simulink model "mcbdemo_28035_TARGET"  (R2021a)
settings: Solver=FixedStepDiscrete  StartTime=0.0  StopTime=4  RelTol=1e-3  EnableMultiTasking=on
InitFcn:
  | mcb_28035_parameters;
values from neighbouring files (symbols this model uses):
  Gain = 10    [mcb_28035_parameters.m]
  T_pwm = 1/PWM_frequency    (= 0.0001)    [mcb_28035_parameters.m]
  Ts = T_pwm    (= 0.0001)    [mcb_28035_parameters.m]
  Ts_inverter = T_pwm/2    (= 5e-05)    [mcb_28035_parameters.m]
  Ts_motor = T_pwm/2    (= 5e-05)    [mcb_28035_parameters.m]
  Ts_simulink = T_pwm/2    (= 5e-05)    [mcb_28035_parameters.m]
undefined symbols (not defined in the file or in its folder): DiscIntNeverNeededParam, Down, GPTRIP1SEL, GPTRIP2SEL, inverter, PI_params, pmsm, target, TZ1, TZ2, Up
libraries: mcbcontrolslib x20, simulink x11, c2802xlib x9, tiiqmathlib x5, c2803xlib x5, mcbpositiondecoderlib x3, c280xlib x2, dspsigops x1, c2000lib x1, autolibpmsmexterior x1
(part 2 of 2)

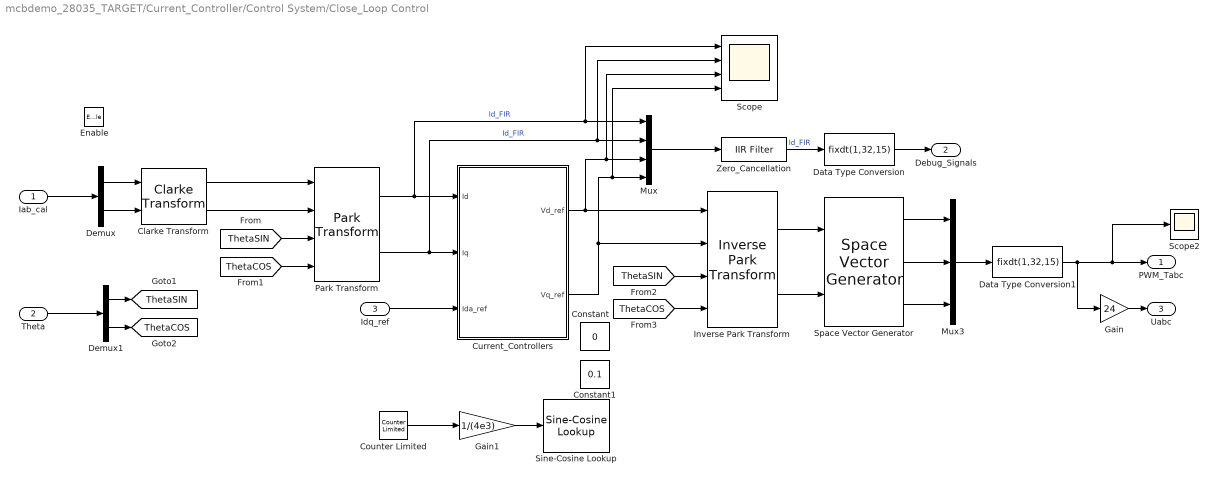
== system mcbdemo_28035_TARGET/Current_Controller/Control System/Close_Loop Control ==
  Iab_cal : Inport
  Theta : Inport  Port=2
  Idq_ref : Inport  Port=3
  Enable : EnablePort
  Clarke Transform : mcbcontrolslib/Clarke Transform  VariantControl=Variant2
  Constant : Constant  Value=0  OutDataTypeStr=fixdt(1,32,24)
  Constant1 : Constant  Value=0.1  OutDataTypeStr=fixdt(1,32,24)
  Counter Limited : simulink/Sources/Counter Limited  uplimit=4e3  tsamp=-1
  Current_Controllers : Subsystem
  Data Type Conversion : DataTypeConversion  OutDataTypeStr=fixdt(1,32,15)
  Data Type Conversion1 : DataTypeConversion  OutDataTypeStr=fixdt(1,32,15)  RndMeth=Simplest
  Demux : Demux  Outputs=2
  Demux1 : Demux  Outputs=2
  Gain : Gain  Gain=24  OutDataTypeStr=Inherit: Same as input
  Gain1 : Gain  Gain=1/(4e3)  OutDataTypeStr=fixdt(1,32,24)
  Inverse Park Transform : mcbcontrolslib/Inverse Park Transform  AxisAlignment=D-axis
  Mux : Mux
  Mux3 : Mux  Inputs=3
  Park Transform : mcbcontrolslib/Park Transform  AxisAlignment=D-axis
      settings: SourceProductBaseCode=MT
  Scope : Scope  NumInputPorts=4
  Scope2 : Scope
  Sine-Cosine Lookup : mcbcontrolslib/Sine-Cosine Lookup  AngleInput=Per-unit  N_points=1024
      settings: SourceProductBaseCode=MT
  Space Vector Generator : mcbcontrolslib/Space Vector Generator
      settings: SourceProductBaseCode=MT
  Zero_Cancellation : mcbcontrolslib/IIR Filter  VariantControl=Low Pass Filter  VariantSelect=Low-pass  Filter_constant=0.001  advancedSettings=on  Ts=1e-4  cutOff_freq=1.5931
      settings: SourceProductBaseCode=MT
  PWM_Tabc : Outport
  Debug_Signals : Outport  Port=2
  Uabc : Outport  Port=3
  tag scope: ThetaCOS=global, ThetaSIN=global
  wires:
  Clarke Transform/1 -> Park Transform/1
  Theta/1 -> Demux1/1
  Iab_cal/1 -> Demux/1
  Inverse Park Transform/2 -> Space Vector Generator/2
  Demux/1 -> Clarke Transform/1
  Space Vector Generator/1 -> Mux3/1
  Space Vector Generator/2 -> Mux3/2
  Data Type Conversion1/1 -> Gain/1, Scope2/1, PWM_Tabc/1
  Idq_ref/1 -> Current_Controllers/3(Ida_ref)
  Demux1/1 -> [ThetaSIN]
  Demux/2 -> Clarke Transform/2
  Demux1/2 -> [ThetaCOS]
  [ThetaCOS] -> Park Transform/4
  [ThetaSIN] -> Park Transform/3
  Clarke Transform/2 -> Park Transform/2
  Current_Controllers/1(Vd_ref) -> Inverse Park Transform/1, Scope/3, Mux/3
  Current_Controllers/2(Vq_ref) -> Inverse Park Transform/2, Scope/4, Mux/4
  Inverse Park Transform/1 -> Space Vector Generator/1
  Space Vector Generator/3 -> Mux3/3
  Mux/1 -> Zero_Cancellation/1
  Park Transform/1 -> Current_Controllers/1(Id), Mux/1, Scope/1  "Id_FIR"
  Park Transform/2 -> Current_Controllers/2(Iq), Scope/2, Mux/2  "Id_FIR"
  Data Type Conversion/1 -> Debug_Signals/1
  Zero_Cancellation/1 -> Data Type Conversion/1  "Id_FIR"
  Mux3/1 -> Data Type Conversion1/1
  Gain/1 -> Uabc/1
  Counter Limited/1 -> Gain1/1
  Gain1/1 -> Sine-Cosine Lookup/1
  [ThetaSIN] -> Inverse Park Transform/3
  [ThetaCOS] -> Inverse Park Transform/4

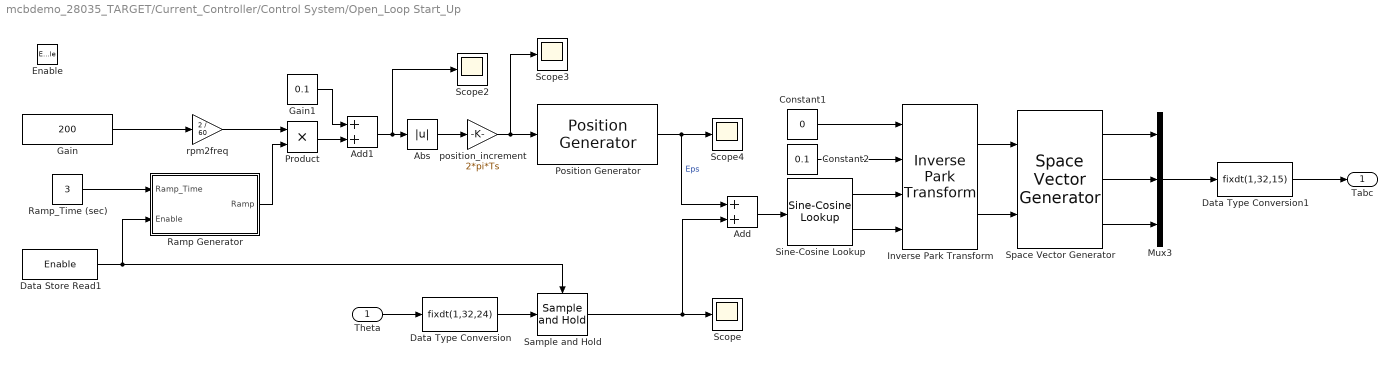
== system mcbdemo_28035_TARGET/Current_Controller/Control System/Open_Loop Start_Up ==
  Theta : Inport
  Enable : EnablePort  StatesWhenEnabling=reset
  Abs : Abs
  Add : Sum
  Add1 : Sum
  Constant1 : Constant  Value=0  OutDataTypeStr=fixdt(1,32,24)
  Constant2 : Constant  Value=0.1  OutDataTypeStr=fixdt(1,32,24)
  Data Store Read1 : DataStoreRead  DataStoreName=Enable  IndexOptions=Index vector (dialog)  Indices=1  OutputSizes=1
  Data Type Conversion : DataTypeConversion  OutDataTypeStr=fixdt(1,32,24)
  Data Type Conversion1 : DataTypeConversion  OutDataTypeStr=fixdt(1,32,15)  RndMeth=Simplest
  Gain : Constant  Value=200  OutDataTypeStr=fixdt(1,32,15)  SampleTime=-1
  Gain1 : Constant  Value=0.1  OutDataTypeStr=fixdt(1,32,24)  SampleTime=-1
  Inverse Park Transform : mcbcontrolslib/Inverse Park Transform  AxisAlignment=D-axis
  Mux3 : Mux  Inputs=3
  Position Generator : mcbcontrolslib/Position Generator  AngleOutput=Radians  ThetaSource=External  ThetaInput=5e-4  DataType=double  ExternalReset=none  Offset=0
      settings: SourceProductBaseCode=MT
  Product : Product  RndMeth=Simplest  OutDataTypeStr=Inherit: Same as first input
  Ramp Generator : Subsystem
  Ramp_Time (sec) : Constant  Value=3  OutDataTypeStr=fixdt(1,32,24)  SampleTime=-1
  Sample and Hold : dspsigops/Sample and Hold  trig=Rising edge  initCond=0  latchinput=off
  Scope{,2..4} (4 alike) : Scope
  Sine-Cosine Lookup : mcbcontrolslib/Sine-Cosine Lookup  AngleInput=Radians  N_points=1024
      settings: SourceProductBaseCode=MT
  Space Vector Generator : mcbcontrolslib/Space Vector Generator
      settings: SourceProductBaseCode=MT
  position_increment : Gain  Gain=2*pi*Ts  RndMeth=Simplest  OutDataTypeStr=Inherit: Same as input
  rpm2freq : Gain  Gain=2 / 60  OutDataTypeStr=fixdt(1,32,24)  RndMeth=Simplest
  Tabc : Outport
  wires:
  Sine-Cosine Lookup/2 -> Inverse Park Transform/4
  Mux3/1 -> Data Type Conversion1/1
  Constant1/1 -> Inverse Park Transform/1
  Inverse Park Transform/2 -> Space Vector Generator/2
  Sine-Cosine Lookup/1 -> Inverse Park Transform/3
  Space Vector Generator/2 -> Mux3/2
  Space Vector Generator/1 -> Mux3/1
  Inverse Park Transform/1 -> Space Vector Generator/1
  Space Vector Generator/3 -> Mux3/3
  Data Type Conversion1/1 -> Tabc/1
  Gain/1 -> rpm2freq/1
  rpm2freq/1 -> Product/1
  Ramp_Time (sec)/1 -> Ramp Generator/1(Ramp_Time)
  Ramp Generator/1(Ramp) -> Product/2
  Data Store Read1/1 -> Sample and Hold/Trigger, Ramp Generator/2(Enable)
  Constant2/1 -> Inverse Park Transform/2
  Abs/1 -> position_increment/1
  Data Type Conversion/1 -> Sample and Hold/1
  Position Generator/1 -> Add/1, Scope4/1  "Eps"
  Add/1 -> Sine-Cosine Lookup/1
  Sample and Hold/1 -> Scope/1, Add/2
  position_increment/1 -> Position Generator/1, Scope3/1
  Product/1 -> Add1/2
  Add1/1 -> Scope2/1, Abs/1
  Gain1/1 -> Add1/1
  Theta/1 -> Data Type Conversion/1

== system mcbdemo_28035_TARGET/Current_Controller/HW_Inputs/Sensor Driver Blocks (codegen) ==
  Sim : Inport
  Mux1 : Mux
  Pos_A : c2802xlib/ADC  blkParamProc=C2000  ADCModule=1  samplingMode=Single sample mode  ADCResolution=12-bit (Single-ended input)  useSOC1=SOC2  useSOC2=SOC0_SOC1  SOCAcquisitionWindow=15  SOCTriggerSource=ePWM1_ADCSOCA  SOCInterruptTrigger=No ADCINT  Ts=-1  dType=uint16  postInterrupt=off  interruptSel=ADCINT1  ADCINTContinuous=on  endma=off  chdma=1  conv1=ADCINA4  conv2=ADCINA0 and ADCINB0  conv1_Type4=ADCIN0  conv2_Type4=ADCIN0 and ADCIN1
  Pos_B : c2802xlib/ADC  blkParamProc=C2000  ADCModule=1  samplingMode=Single sample mode  ADCResolution=12-bit (Single-ended input)  useSOC1=SOC3  useSOC2=SOC0_SOC1  SOCAcquisitionWindow=15  SOCTriggerSource=ePWM1_ADCSOCA  SOCInterruptTrigger=No ADCINT  Ts=-1  dType=uint16  postInterrupt=off  interruptSel=ADCINT1  ADCINTContinuous=on  endma=off  chdma=1  conv1=ADCINA3  conv2=ADCINA0 and ADCINB0  conv1_Type4=ADCIN0  conv2_Type4=ADCIN0 and ADCIN1
  SO1_CurrentA : c2802xlib/ADC  blkParamProc=C2000  ADCModule=1  samplingMode=Single sample mode  ADCResolution=12-bit (Single-ended input)  useSOC1=SOC0  useSOC2=SOC0_SOC1  SOCAcquisitionWindow=15  SOCTriggerSource=ePWM1_ADCSOCA  SOCInterruptTrigger=No ADCINT  Ts=-1  dType=uint16  postInterrupt=off  interruptSel=ADCINT1  ADCINTContinuous=on  endma=off  chdma=1  conv1=ADCINA7  conv2=ADCINA0 and ADCINB0  conv1_Type4=ADCIN0  conv2_Type4=ADCIN0 and ADCIN1
  SO2_CurrentB : c2802xlib/ADC  blkParamProc=C2000  ADCModule=1  samplingMode=Single sample mode  ADCResolution=12-bit (Single-ended input)  useSOC1=SOC1  useSOC2=SOC0_SOC1  SOCAcquisitionWindow=15  SOCTriggerSource=ePWM2_ADCSOCA  SOCInterruptTrigger=No ADCINT  Ts=-1  dType=uint16  postInterrupt=on  interruptSel=ADCINT2  ADCINTContinuous=on  endma=off  chdma=1  conv1=ADCINA6  conv2=ADCINA0 and ADCINB0  conv1_Type4=ADCIN0  conv2_Type4=ADCIN0 and ADCIN1
  Terminator : Terminator
  Out : Outport
  wires:
  Mux1/1 -> Out/1
  Pos_A/1 -> Mux1/3
  SO2_CurrentB/1 -> Mux1/2
  Pos_B/1 -> Mux1/4
  SO1_CurrentA/1 -> Mux1/1
  Sim/1 -> Terminator/1

== system mcbdemo_28035_TARGET/Current_Controller/HW_Inputs/Sensor Driver Blocks (sim) ==
  Sim : Inport
  Out : Outport
  wires:
  Sim/1 -> Out/1

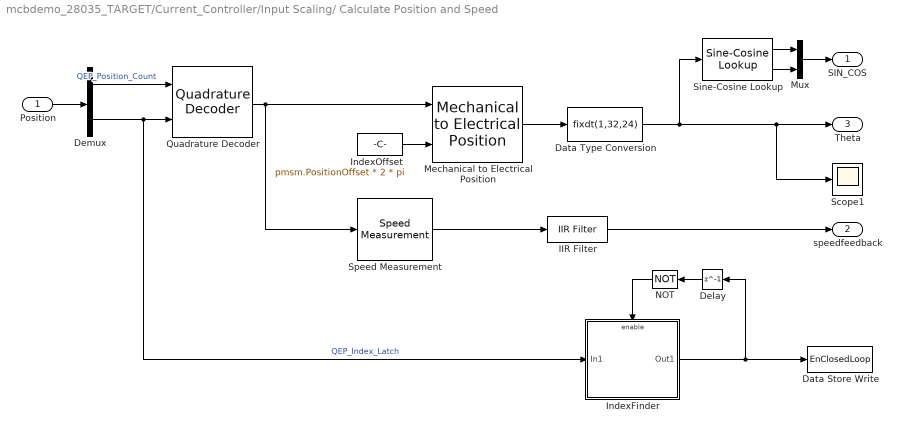
== system mcbdemo_28035_TARGET/Current_Controller/Input Scaling/ Calculate Position and Speed ==
  Position : Inport
  Data Store Write : DataStoreWrite  DataStoreName=EnClosedLoop  IndexOptions=Index vector (dialog)  Indices=1  OutputSizes=1
  Data Type Conversion : DataTypeConversion  OutDataTypeStr=fixdt(1,32,24)
  Delay : Delay  DelayLength=1
  Demux : Demux  Outputs=2
  IIR Filter : mcbcontrolslib/IIR Filter  VariantControl=Low Pass Filter  VariantSelect=Low-pass  Filter_constant=0.01  advancedSettings=off  Ts=50e-6  cutOff_freq=32.1525
      settings: SourceProductBaseCode=MT
  IndexFinder : Subsystem
  IndexOffset : Constant  Value=pmsm.PositionOffset * 2 * pi  OutDataTypeStr=fixdt(1,32,15)  SampleTime=-1
  Mechanical to Electrical Position : mcbpositiondecoderlib/Mechanical to Electrical Position  NrPP=pmsm.p  selectedRange=Radians  MechOfstInputType=Input port  mechOffsetIn=0  maxAngleIn=2*pi  InputDataType=fixdt(1,32,15)  VariantSelect=floating-point
      settings: SourceProductBaseCode=MT
  Mux : Mux  Inputs=2
  NOT : Logic  Operator=NOT  AllPortsSameDT=off  OutDataTypeStr=boolean
  Quadrature Decoder : mcbpositiondecoderlib/Quadrature Decoder  EncoderSlitsPerRevolution=pmsm.QEPSlits  EncoderCountsPerSlit=4  CounterSize=16 bits  ExternalIndexCount=on  PositionUnit=Radians  PositionDataType=fixdt(1,32,15)
      settings: SourceProductBaseCode=MT
  Scope1 : Scope
  Sine-Cosine Lookup : mcbcontrolslib/Sine-Cosine Lookup  AngleInput=Radians  N_points=1024
      settings: SourceProductBaseCode=MT
  Speed Measurement : mcbpositiondecoderlib/Speed Measurement  PositionUnit=Radians  SpeedCalculationMode=Time interval for speed calculation  SampleTimeAsync=Ts  MaximumApplicationSpeed=6000  SpeedResolution=5e-6  DelayLength=20  MaximumMeasurableSpeed=14999  MeasurableSpeedResolution=6.9849e-06  SpeedUnit=Radians/Sec  PerUnitSpeed=PU_System.N_base  SpeedDataType=fixdt(1,32,15)
      settings: SourceProductBaseCode=MT
  SIN_COS : Outport  VectorParamsAs1DForOutWhenUnconnected=off
  speedfeedback : Outport  Port=2  VectorParamsAs1DForOutWhenUnconnected=off
  Theta : Outport  Port=3  VectorParamsAs1DForOutWhenUnconnected=off
  wires:
  Speed Measurement/1 -> IIR Filter/1
  Mechanical to Electrical Position/1 -> Data Type Conversion/1
  Demux/1 -> Quadrature Decoder/1  "QEP_Position_Count"
  Quadrature Decoder/1 -> Mechanical to Electrical Position/1, Speed Measurement/1
  IIR Filter/1 -> speedfeedback/1
  Delay/1 -> NOT/1
  NOT/1 -> IndexFinder/Enable
  IndexFinder/1(Out1) -> Data Store Write/1, Delay/1
  Demux/2 -> Quadrature Decoder/2, IndexFinder/1(In1)  "QEP_Index_Latch"
  Position/1 -> Demux/1
  IndexOffset/1 -> Mechanical to Electrical Position/2
  Sine-Cosine Lookup/2 -> Mux/2
  Sine-Cosine Lookup/1 -> Mux/1
  Mux/1 -> SIN_COS/1
  Data Type Conversion/1 -> Sine-Cosine Lookup/1, Scope1/1, Theta/1

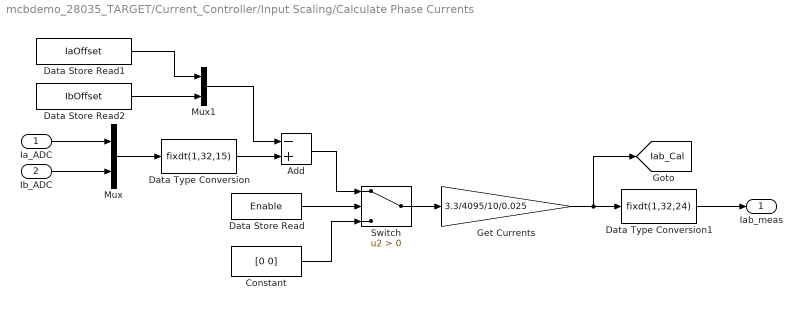
== system mcbdemo_28035_TARGET/Current_Controller/Input Scaling/Calculate Phase Currents ==
  Ia_ADC : Inport
  Ib_ADC : Inport  Port=2
  Add : Sum  Inputs=-+
  Constant : Constant  Value=[0 0]  OutDataTypeStr=fixdt(1,32,15)
  Data Store Read : DataStoreRead  DataStoreName=Enable  IndexOptions=Index vector (dialog)  Indices=1  OutputSizes=1
  Data Store Read1 : DataStoreRead  DataStoreName=IaOffset  IndexOptions=Index vector (dialog)  Indices=1  OutputSizes=1
  Data Store Read2 : DataStoreRead  DataStoreName=IbOffset  IndexOptions=Index vector (dialog)  Indices=1  OutputSizes=1
  Data Type Conversion : DataTypeConversion  OutDataTypeStr=fixdt(1,32,15)  RndMeth=Simplest
  Data Type Conversion1 : DataTypeConversion  OutDataTypeStr=fixdt(1,32,24)  RndMeth=Simplest
  Get Currents : Gain  Gain=3.3/4095/10/0.025  RndMeth=Simplest  OutDataTypeStr=Inherit: Same as input
  Mux : Mux  Inputs=2
  Mux1 : Mux  Inputs=2
  Switch : Switch  Criteria=u2 > Threshold
  Iab_meas : Outport  VectorParamsAs1DForOutWhenUnconnected=off
  tag scope: Iab_Cal=global
  wires:
  Data Type Conversion/1 -> Add/2
  Ia_ADC/1 -> Mux/1
  Ib_ADC/1 -> Mux/2
  Mux/1 -> Data Type Conversion/1
  Data Store Read1/1 -> Mux1/1
  Data Store Read2/1 -> Mux1/2
  Mux1/1 -> Add/1
  Get Currents/1 -> Data Type Conversion1/1, [Iab_Cal]
  Data Type Conversion1/1 -> Iab_meas/1
  Data Store Read/1 -> Switch/2
  Add/1 -> Switch/1
  Switch/1 -> Get Currents/1
  Constant/1 -> Switch/3

== system mcbdemo_28035_TARGET/Current_Controller/Input Scaling/Calculate Phase Currents1 ==
  Position : Inport
  Add : Sum  Inputs=-+
  Data Store Read1 : DataStoreRead  DataStoreName=PosaOffset  IndexOptions=Index vector (dialog)  Indices=1  OutputSizes=1
  Data Store Read2 : DataStoreRead  DataStoreName=PosbOffset  IndexOptions=Index vector (dialog)  Indices=1  OutputSizes=1
  Data Type Conversion : DataTypeConversion  OutDataTypeStr=fixdt(1,32,15)  RndMeth=Simplest
  Gain2 : Gain  OutDataTypeStr=Inherit: Same as input
  Mux1 : Mux  Inputs=2
  Posab_meas : Outport  VectorParamsAs1DForOutWhenUnconnected=off
  tag scope: PosAB=global
  wires:
  Data Type Conversion/1 -> Add/2
  Data Store Read1/1 -> Mux1/1
  Data Store Read2/1 -> Mux1/2
  Gain2/1 -> Posab_meas/1
  Add/1 -> [PosAB], Gain2/1
  Mux1/1 -> Add/1
  Position/1 -> Data Type Conversion/1

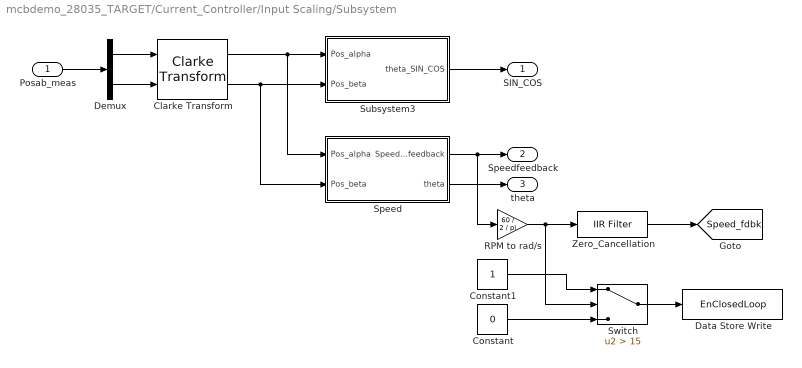
== system mcbdemo_28035_TARGET/Current_Controller/Input Scaling/Subsystem ==
  Posab_meas : Inport
  Clarke Transform : mcbcontrolslib/Clarke Transform  VariantControl=Variant2
  Constant : Constant  Value=0  OutDataTypeStr=boolean
  Constant1 : Constant  OutDataTypeStr=boolean
  Data Store Write : DataStoreWrite  DataStoreName=EnClosedLoop  IndexOptions=Index vector (dialog)  Indices=1  OutputSizes=1
  Demux : Demux  Outputs=2
  RPM to rad/s : Gain  Gain=60 / 2 / pi  RndMeth=Simplest  OutDataTypeStr=Inherit: Same as input
  Speed : Subsystem
  Subsystem3 : Subsystem
  Switch : Switch  Criteria=u2 > Threshold  Threshold=15
  Zero_Cancellation : mcbcontrolslib/IIR Filter  VariantControl=Low Pass Filter  VariantSelect=Low-pass  Filter_constant=0.001  advancedSettings=on  Ts=1e-4  cutOff_freq=1.5931
      settings: SourceProductBaseCode=MT
  SIN_COS : Outport
  Speedfeedback : Outport  Port=2
  theta : Outport  Port=3
  tag scope: Speed_fdbk=global
  wires:
  Clarke Transform/2 -> Subsystem3/2(Pos_beta), Speed/2(Pos_beta)
  Clarke Transform/1 -> Subsystem3/1(Pos_alpha), Speed/1(Pos_alpha)
  Speed/1(Speed_feedback) -> RPM to rad/s/1, Speedfeedback/1
  Demux/1 -> Clarke Transform/1
  Demux/2 -> Clarke Transform/2
  Subsystem3/1(theta_SIN_COS) -> SIN_COS/1
  Posab_meas/1 -> Demux/1
  RPM to rad/s/1 -> Zero_Cancellation/1, Switch/2
  Constant/1 -> Switch/3
  Constant1/1 -> Switch/1
  Zero_Cancellation/1 -> [Speed_fdbk]
  Speed/2(theta) -> theta/1
  Switch/1 -> Data Store Write/1

== system mcbdemo_28035_TARGET/Current_Controller/PWM_output (Code Generation)/PWM scaling ==
  in : Inport
  Add : Sum
  Constant : Constant  OutDataTypeStr=fixdt(1,32,15)  SampleTime=-1
  Data Type Conversion1 : DataTypeConversion  OutDataTypeStr=uint16
  IQN x IQN : tiiqmathlib/IQN x IQN  multiplyOption=Multiply
      settings: SourceProductBaseCode=TIC2000
  Map to 2 : Constant  Value=1500  OutDataTypeStr=fixdt(1,32,15)  SampleTime=-1
  Saturation : Saturate  UpperLimit=2999  LowerLimit=1
  Out1 : Outport  VectorParamsAs1DForOutWhenUnconnected=off
  wires:
  Map to 2/1 -> IQN x IQN/2
  Constant/1 -> Add/1
  Add/1 -> IQN x IQN/1
  Data Type Conversion1/1 -> Out1/1
  IQN x IQN/1 -> Saturation/1
  in/1 -> Add/2
  Saturation/1 -> Data Type Conversion1/1

== system mcbdemo_28035_TARGET/Current_Controller/SCI_TX(Code Generation)/SCI (Code Generation) ==
  Iab_meas : Inport
  Trigger : TriggerPort  TriggerType=falling  VariantControl=(inherit)  PortDimensions=1
  Data Type Conversion : DataTypeConversion  OutDataTypeStr=int32  RndMeth=Simplest
  Data Type Conversion3 : DataTypeConversion  OutDataTypeStr=uint32  RndMeth=Simplest
  Data_Logging : Subsystem
  Demux2 : Demux  Outputs=2
  While Iterator Subsystem : Subsystem  TreatAsAtomicUnit=on
  wires:
  Demux2/2 -> While Iterator Subsystem/2(Iteration)  "SCI_Tx_Iteration"
  Demux2/1 -> While Iterator Subsystem/1(Data)  "SCI_Tx_Data"
  Data_Logging/1(SCI_Tx) -> Demux2/1
  Data Type Conversion3/1 -> Data_Logging/1(Data_Log)
  Iab_meas/1 -> Data Type Conversion/1
  Data Type Conversion/1 -> Data Type Conversion3/1

== system mcbdemo_28035_TARGET/Inverter and Motor - Plant Model/Simulation/Inverter ==
  Duty_abc : Inport
  Average_Value_Inverter : Subsystem
  Constant2 : Constant  Value=inverter.V_dc  OutDataTypeStr=single  SampleTime=-1
  Data Type Conversion1 : DataTypeConversion  OutDataTypeStr=single  RndMeth=Simplest
  Demux : Demux  Outputs=3
  Inverter_delay : DiscreteTransferFcn  Numerator=[1-exp(-Ts_inverter/(T_pwm/2))]  Denominator=[1 -exp(-Ts_inverter/(T_pwm/2))]  RndMeth=Simplest
  Mux : Mux  Inputs=3
  Rate Transition3 : RateTransition  Integrity=off  OutPortSampleTime=Ts_inverter
  Vabc : Outport  VectorParamsAs1DForOutWhenUnconnected=off
  wires:
  Average_Value_Inverter/2(Vb) -> Mux/2
  Mux/1 -> Inverter_delay/1  "Vabc"
  Constant2/1 -> Average_Value_Inverter/4(Vdc)
  Average_Value_Inverter/3(Vc) -> Mux/3
  Average_Value_Inverter/1(Va) -> Mux/1
  Demux/1 -> Average_Value_Inverter/1(Vao)
  Demux/3 -> Average_Value_Inverter/3(Vco)
  Demux/2 -> Average_Value_Inverter/2(Vbo)
  Data Type Conversion1/1 -> Rate Transition3/1
  Rate Transition3/1 -> Demux/1
  Inverter_delay/1 -> Vabc/1
  Duty_abc/1 -> Data Type Conversion1/1

== system mcbdemo_28035_TARGET/Inverter and Motor - Plant Model/Simulation/Load_Profile (Torque) ==
  Data Type Conversion : DataTypeConversion  OutDataTypeStr=single
  IIR Filter : mcbcontrolslib/IIR Filter  VariantControl=Low Pass Filter  VariantSelect=Low-pass  Filter_constant=0.01  advancedSettings=off  Ts=50e-6  cutOff_freq=32.1525
      settings: SourceProductBaseCode=MT
  T_load : Step  Time=2  Before=0.05*pmsm.T_rated  After=0.5*pmsm.T_rated  SampleTime=Ts_simulink
  Load_Trq : Outport  VectorParamsAs1DForOutWhenUnconnected=off
  wires:
  Data Type Conversion/1 -> IIR Filter/1
  T_load/1 -> Data Type Conversion/1
  IIR Filter/1 -> Load_Trq/1

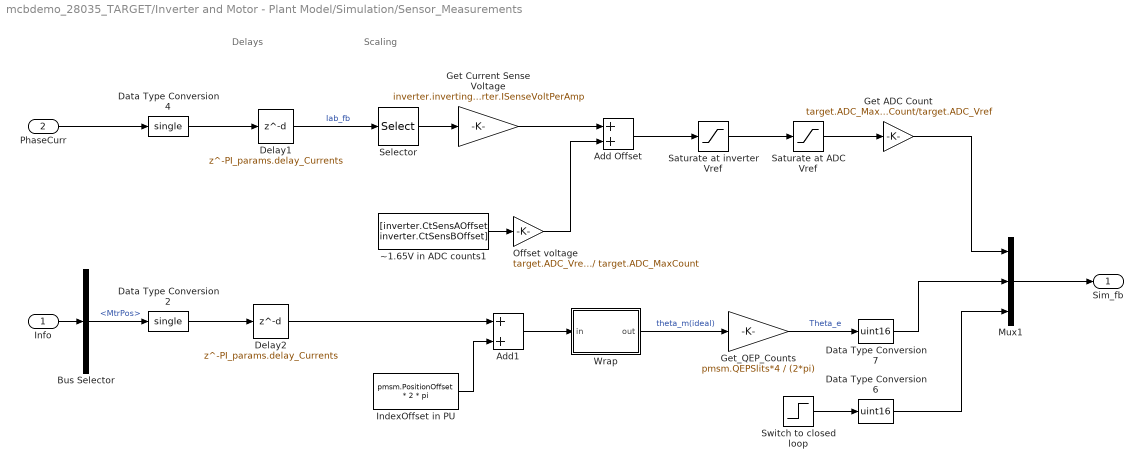
== system mcbdemo_28035_TARGET/Inverter and Motor - Plant Model/Simulation/Sensor_Measurements ==
  note: Scaling
  note: Delays
  Info : Inport
  PhaseCurr : Inport  Port=2
  Add Offset : Sum  RndMeth=Simplest
  Add1 : Sum  RndMeth=Simplest
  Bus Selector : BusSelector  OutputSignals=MtrPos
  Data Type Conversion2 : DataTypeConversion  OutDataTypeStr=single  RndMeth=Simplest
  Data Type Conversion4 : DataTypeConversion  OutDataTypeStr=single  RndMeth=Simplest
  Data Type Conversion6 : DataTypeConversion  OutDataTypeStr=uint16  RndMeth=Simplest
  Data Type Conversion7 : DataTypeConversion  OutDataTypeStr=uint16  RndMeth=Simplest
  Delay1 : Delay  DelayLength=PI_params.delay_Currents
  Delay2 : Delay  DelayLength=PI_params.delay_Currents
  Get ADC Count : Gain  Gain=target.ADC_MaxCount/target.ADC_Vref  OutMin=0  OutMax=target.ADC_MaxCount  OutDataTypeStr=uint16  RndMeth=Simplest
  Get Current Sense Voltage : Gain  Gain=inverter.invertingAmp * inverter.ISenseVoltPerAmp  RndMeth=Simplest  OutDataTypeStr=Inherit: Same as input
  Get_QEP_Counts : Gain  Gain=pmsm.QEPSlits*4 / (2*pi)  RndMeth=Simplest
  IndexOffset in PU : Constant  Value=pmsm.PositionOffset * 2 * pi  OutDataTypeStr=single  SampleTime=-1
  Mux1 : Mux  Inputs=3
  Offset voltage : Gain  Gain=target.ADC_Vref / target.ADC_MaxCount  RndMeth=Simplest
  Saturate at ADC Vref : Saturate  UpperLimit=target.ADC_Vref  LowerLimit=0
  Saturate at inverter Vref : Saturate  UpperLimit=inverter.ISenseVref  LowerLimit=0
  Selector : Selector  InputPortWidth=3  IndexOptions=Index vector (dialog)  Indices=[1 2]  OutputSizes=1
  Switch to closed loop : Step  Time=0.1  SampleTime=Ts_motor
  Wrap : Subsystem
  ~1.65V in ADC counts1 : Constant  Value=[inverter.CtSensAOffset inverter.CtSensBOffset]  OutDataTypeStr=uint16  SampleTime=-1
  Sim_fb : Outport  VectorParamsAs1DForOutWhenUnconnected=off
  wires:
  Delay1/1 -> Selector/1  "Iab_fb"
  Data Type Conversion4/1 -> Delay1/1
  PhaseCurr/1 -> Data Type Conversion4/1
  Info/1 -> Bus Selector/1
  Bus Selector/1 -> Data Type Conversion2/1  "<MtrPos>"
  Data Type Conversion2/1 -> Delay2/1
  Delay2/1 -> Add1/1
  IndexOffset in PU/1 -> Add1/2
  Add1/1 -> Wrap/1(in)
  Get_QEP_Counts/1 -> Data Type Conversion7/1  "Theta_e"
  Wrap/1(out) -> Get_QEP_Counts/1  "theta_m(ideal)"
  Switch to closed loop/1 -> Data Type Conversion6/1
  ~1.65V in ADC counts1/1 -> Offset voltage/1
  Get Current Sense Voltage/1 -> Add Offset/1
  Saturate at ADC Vref/1 -> Get ADC Count/1
  Add Offset/1 -> Saturate at inverter Vref/1
  Saturate at inverter Vref/1 -> Saturate at ADC Vref/1
  Selector/1 -> Get Current Sense Voltage/1
  Offset voltage/1 -> Add Offset/2
  Data Type Conversion6/1 -> Mux1/3
  Data Type Conversion7/1 -> Mux1/2
  Get ADC Count/1 -> Mux1/1
  Mux1/1 -> Sim_fb/1

== system mcbdemo_28035_TARGET/Serial Receive/Simulation/Parse ==
  Enable_PWM : Inport
  Debug_signals : Inport  Port=2
  Bitwise Operator : simulink/Logic and Bit Operations/Bitwise Operator  logicop=AND  UseBitMask=on  BitMask=hex2dec('0001')  BitMaskRealWorld=Stored Integer
  Bitwise Operator1 : simulink/Logic and Bit Operations/Bitwise Operator  logicop=AND  UseBitMask=on  BitMask=hex2dec('00F0')  BitMaskRealWorld=Stored Integer
  Shift Arithmetic1 : ArithShift  BitShiftNumber=-4
  Sum : Sum
  Data : Outport
  wires:
  Bitwise Operator/1 -> Sum/1
  Debug_signals/1 -> Shift Arithmetic1/1
  Sum/1 -> Data/1
  Shift Arithmetic1/1 -> Bitwise Operator1/1
  Enable_PWM/1 -> Bitwise Operator/1
  Bitwise Operator1/1 -> Sum/2

== system mcbdemo_28035_TARGET/Current_Controller/Control System/Close_Loop Control/Current_Controllers ==
  Id : Inport
  Iq : Inport  Port=2
  Ida_ref : Inport  Port=3
  DQ Limiter : mcbcontrolslib/DQ Limiter  Vmax=0.95
      settings: SourceProductBaseCode=MT
  Demux : Demux  Outputs=2
  PI_Controller_Id : Subsystem
  PI_Controller_Iq : Subsystem
  Terminator : Terminator
  Vd_ref : Outport  VectorParamsAs1DForOutWhenUnconnected=off
  Vq_ref : Outport  Port=2  VectorParamsAs1DForOutWhenUnconnected=off
  wires:
  Iq/1 -> PI_Controller_Iq/2(I_fb)  "Iq_fb"
  Id/1 -> PI_Controller_Id/2(I_fb)  "Id_fb"
  Demux/1 -> PI_Controller_Id/1(I_ref)  "Id_Ref"
  Demux/2 -> PI_Controller_Iq/1(I_ref)  "Iq_Ref"
  Ida_ref/1 -> Demux/1
  PI_Controller_Id/1(V_ref) -> DQ Limiter/1
  PI_Controller_Iq/1(V_ref) -> DQ Limiter/2
  DQ Limiter/2 -> Vq_ref/1
  DQ Limiter/1 -> Vd_ref/1
  DQ Limiter/3 -> Terminator/1

== system mcbdemo_28035_TARGET/Current_Controller/Control System/Open_Loop Start_Up/Ramp Generator ==
  Ramp_Time : Inport
  Enable : Inport  Port=2
  Divide : Product  Inputs=*/  RndMeth=Simplest  OutDataTypeStr=Inherit: Same as first input
  NOT : Logic  Operator=NOT  IconShape=distinctive  AllPortsSameDT=off  OutDataTypeStr=boolean
  One : Constant  OutDataTypeStr=fixdt(1,32,24)  SampleTime=-1
  Ramp Generator : DiscreteIntegrator  IntegratorMethod=Accumulation: Forward Euler  gainval=1  ExternalReset=sampled level  SampleTime=-1  OutDataTypeStr=fixdt(1,32,24)  RndMeth=Simplest  LimitOutput=on  UpperSaturationLimit=1  LowerSaturationLimit=0  ICPrevOutput=DiscIntNeverNeededParam  ICPrevScaledInput=DiscIntNeverNeededParam
  Sample_Time : Gain  Gain=Ts  RndMeth=Simplest  OutDataTypeStr=Inherit: Same as input
  Ramp : Outport
  wires:
  Divide/1 -> Sample_Time/1
  Ramp Generator/1 -> Ramp/1  "Eps"
  Sample_Time/1 -> Ramp Generator/1
  One/1 -> Divide/1
  Ramp_Time/1 -> Divide/2
  Enable/1 -> NOT/1
  NOT/1 -> Ramp Generator/2

== system mcbdemo_28035_TARGET/Current_Controller/Input Scaling/ Calculate Position and Speed/IndexFinder ==
  In1 : Inport
  Enable : EnablePort
  AND : Logic  AllPortsSameDT=off  OutDataTypeStr=boolean
  Compare To Constant : simulink/Logic and Bit Operations/Compare To Constant  relop===  const=0  OutDataTypeStr=boolean
  Compare To Constant1 : simulink/Logic and Bit Operations/Compare To Constant  relop=>  const=0  OutDataTypeStr=boolean
  Delay3 : Delay  DelayLength=1
  Out1 : Outport
  wires:
  In1/1 -> Delay3/1, Compare To Constant1/1
  Compare To Constant1/1 -> AND/2
  Compare To Constant/1 -> AND/1
  Delay3/1 -> Compare To Constant/1
  AND/1 -> Out1/1

== system mcbdemo_28035_TARGET/Current_Controller/Input Scaling/Subsystem/Speed ==
  Pos_alpha : Inport
  Pos_beta : Inport  Port=2
  Add3 : Sum  OutDataTypeStr=fixdt(1,32,15)  RndMeth=Simplest
  Arctangent IQN1 : tiiqmathlib/Arctangent IQN  tanOption=atan2PU (per unit)
      settings: SourceProductBaseCode=TIC2000
  Data Store Read : DataStoreRead  DataStoreName=ThetaOffset  IndexOptions=Index vector (dialog)  Indices=1  OutputSizes=1
  speed cal : Subsystem
  theta_unify : Subsystem
  Speed_feedback : Outport
  theta : Outport  Port=2
  tag scope: theta=global
  wires:
  theta_unify/1(unified_theta) -> theta/1, [theta], speed cal/1(Theta)
  Data Store Read/1 -> Add3/2
  Arctangent IQN1/1 -> Add3/1
  Pos_alpha/1 -> Arctangent IQN1/1
  Add3/1 -> theta_unify/1(raw_theta)
  Pos_beta/1 -> Arctangent IQN1/2
  speed cal/1(Speed) -> Speed_feedback/1

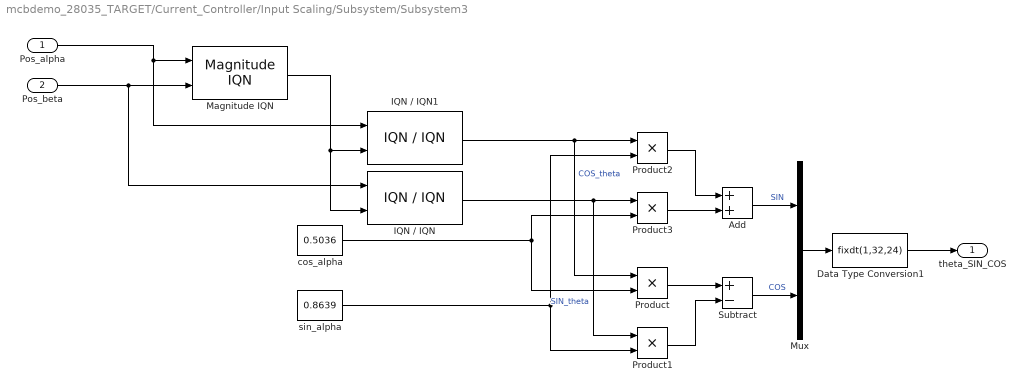
== system mcbdemo_28035_TARGET/Current_Controller/Input Scaling/Subsystem/Subsystem3 ==
  Pos_alpha : Inport
  Pos_beta : Inport  Port=2
  Add : Sum
  Data Type Conversion1 : DataTypeConversion  OutDataTypeStr=fixdt(1,32,24)  RndMeth=Simplest
  IQN / IQN : tiiqmathlib/IQN // IQN
      settings: SourceProductBaseCode=TIC2000
  IQN / IQN1 : tiiqmathlib/IQN // IQN
      settings: SourceProductBaseCode=TIC2000
  Magnitude IQN : tiiqmathlib/Magnitude IQN
      settings: SourceProductBaseCode=TIC2000
  Mux : Mux  Inputs=2
  Product{,1..3} (4 alike) : Product  OutDataTypeStr=Inherit: Same as first input
  Subtract : Sum  Inputs=+-
  cos_alpha : Constant  Value=0.5036  OutDataTypeStr=fixdt(1,32,15)
  sin_alpha : Constant  Value=0.8639  OutDataTypeStr=fixdt(1,32,15)
  theta_SIN_COS : Outport  VectorParamsAs1DForOutWhenUnconnected=off
  wires:
  Pos_alpha/1 -> IQN / IQN1/1, Magnitude IQN/1
  Pos_beta/1 -> IQN / IQN/1, Magnitude IQN/2
  IQN / IQN/1 -> Product1/1, Product3/1  "SIN_theta"
  IQN / IQN1/1 -> Product2/1, Product/1  "COS_theta"
  Magnitude IQN/1 -> IQN / IQN/2, IQN / IQN1/2
  cos_alpha/1 -> Product/2, Product3/2
  sin_alpha/1 -> Product2/2, Product1/2
  Product/1 -> Subtract/1
  Product1/1 -> Subtract/2
  Product3/1 -> Add/2
  Product2/1 -> Add/1
  Add/1 -> Mux/1  "SIN"
  Subtract/1 -> Mux/2  "COS"
  Mux/1 -> Data Type Conversion1/1
  Data Type Conversion1/1 -> theta_SIN_COS/1

== system mcbdemo_28035_TARGET/Current_Controller/SCI_TX(Code Generation)/SCI (Code Generation)/Data_Logging ==
  note: Fast Serial Data Monitoring (32-bit)
  Data_Log : Inport
  Counter Limited : simulink/Sources/Counter Limited  uplimit=100-1  tsamp=-1
  Data : Subsystem  TreatAsAtomicUnit=on
  End : Subsystem  TreatAsAtomicUnit=on
  If : If  IfExpression=u1 == 0  ElseIfExpressions=u1 == 99
  Merge : Merge  Inputs=3
  Merge1 : Merge  Inputs=3
  Mux : Mux  Inputs=2
  Start : Subsystem  TreatAsAtomicUnit=on
  Width : Width  OutDataTypeMode=All ports same datatype  DataType=uint16
  SCI_Tx : Outport
  wires:
  If/3 -> Data/Action
  Data/1(Data_out) -> Merge/3
  Width/1 -> Data/2(Data_width), Start/2(Data_width), End/2(Data_width)
  Merge/1 -> Mux/1  "SCI_Tx_Data"
  Counter Limited/1 -> If/1
  Start/2(Iteration) -> Merge1/1
  Start/1(Data_out) -> Merge/1
  If/2 -> End/Action
  Merge1/1 -> Mux/2  "SCI_Tx_Iteration"
  If/1 -> Start/Action
  End/1(Data_out) -> Merge/2
  End/2(Iteration) -> Merge1/2
  Data/2(Iteration) -> Merge1/3
  Mux/1 -> SCI_Tx/1
  Data_Log/1 -> Start/1(Data), End/1(Data), Data/1(Data), Width/1

== system mcbdemo_28035_TARGET/Current_Controller/SCI_TX(Code Generation)/SCI (Code Generation)/While Iterator Subsystem ==
  Data : Inport
  Iteration : Inport  Port=2
  Add : Sum  Inputs=+-  OutDataTypeStr=Inherit: Same as first input
  Index Vector : MultiPortSwitch  Inputs=1
  SCI Transmit : c280xlib/SCI Transmit  sciModule=A  dataHead=''  dataTail=''  postInterrupt=off  numFifo=1
  While Iterator : WhileIterator  MaxIters=-1  WhileBlockType=do-while  ShowIterationPort=on  OutputDataType=int16
  wires:
  While Iterator/1 -> Add/2, Index Vector/1
  Data/1 -> Index Vector/2
  Index Vector/1 -> SCI Transmit/1
  Add/1 -> While Iterator/1
  Iteration/1 -> Add/1

== system mcbdemo_28035_TARGET/Inverter and Motor - Plant Model/Simulation/Inverter/Average_Value_Inverter ==
  Vao : Inport
  Vbo : Inport  Port=2
  Vco : Inport  Port=3
  Vdc : Inport  Port=4
  Gain : Gain  Gain=1/3  RndMeth=Simplest  OutDataTypeStr=Inherit: Same as input
  Product : Product  RndMeth=Simplest  OutDataTypeStr=Inherit: Same as first input
  Product1 : Product  RndMeth=Simplest  OutDataTypeStr=Inherit: Same as first input
  Product2 : Product  RndMeth=Simplest  OutDataTypeStr=Inherit: Same as first input
  Sum1 : Sum  Inputs=|++--  RndMeth=Simplest  OutDataTypeStr=Inherit: Same as first input
  Sum2 : Sum  Inputs=|++--  RndMeth=Simplest  OutDataTypeStr=Inherit: Same as first input
  Sum3 : Sum  Inputs=|++--  RndMeth=Simplest  OutDataTypeStr=Inherit: Same as first input
  Va : Outport  VectorParamsAs1DForOutWhenUnconnected=off
  Vb : Outport  Port=2  VectorParamsAs1DForOutWhenUnconnected=off
  Vc : Outport  Port=3  VectorParamsAs1DForOutWhenUnconnected=off
  wires:
  Product1/1 -> Vb/1  "Vb"
  Gain/1 -> Product/2, Product1/2, Product2/2
  Sum2/1 -> Product2/1
  Vao/1 -> Sum3/1, Sum3/2, Sum1/4, Sum2/3
  Product2/1 -> Vc/1  "Vb"
  Sum1/1 -> Product1/1
  Vdc/1 -> Gain/1
  Sum3/1 -> Product/1
  Product/1 -> Va/1  "Va"
  Vco/1 -> Sum3/4, Sum1/3, Sum2/2, Sum2/1
  Vbo/1 -> Sum1/1, Sum1/2, Sum3/3, Sum2/4

== system mcbdemo_28035_TARGET/Inverter and Motor - Plant Model/Simulation/Sensor_Measurements/Wrap ==
  in : Inport
  Constant2 : Constant  Value=2*pi  OutDataTypeStr=single  SampleTime=-1
  Mod : Math  Operator=mod  SaturateOnIntegerOverflow=on
  out : Outport  VectorParamsAs1DForOutWhenUnconnected=off
  wires:
  in/1 -> Mod/1
  Constant2/1 -> Mod/2
  Mod/1 -> out/1

== system mcbdemo_28035_TARGET/Current_Controller/Control System/Close_Loop Control/Current_Controllers/PI_Controller_Id ==
  I_ref : Inport
  I_fb : Inport  Port=2
  Data Store Read1 : DataStoreRead  DataStoreName=Enable  IndexOptions=Index vector (dialog)  Indices=1  OutputSizes=1
  Discrete PI Controller with anti-windup & reset : mcbcontrolslib/Discrete PI Controller  with anti-windup & reset  UpperSaturationLimit=0.9*Gain  LowerSaturationLimit=-0.9*Gain
      settings: SourceProductBaseCode=MT
  Gain : Gain  Gain=Gain  OutDataTypeStr=Inherit: Same as input
  Gain1 : Gain  Gain=1/Gain  OutDataTypeStr=Inherit: Same as input
  Ki : Constant  Value=0.0005  OutDataTypeStr=fixdt(1,32,24)  SampleTime=-1
  Ki1 : Constant  Value=0  OutDataTypeStr=fixdt(1,32,24)  SampleTime=-1
  Kp : Constant  Value=0.4  OutDataTypeStr=fixdt(1,32,24)  SampleTime=-1
  Logical Operator : Logic  Operator=NOT  IconShape=distinctive  AllPortsSameDT=off  OutDataTypeStr=boolean
  Sum : Sum  Inputs=|+-  OutDataTypeStr=Inherit: Same as first input
  V_ref : Outport  VectorParamsAs1DForOutWhenUnconnected=off
  wires:
  I_ref/1 -> Sum/1
  I_fb/1 -> Sum/2
  Data Store Read1/1 -> Logical Operator/1
  Discrete PI Controller with anti-windup & reset/1 -> Gain1/1
  Sum/1 -> Gain/1
  Logical Operator/1 -> Discrete PI Controller with anti-windup & reset/4
  Ki1/1 -> Discrete PI Controller with anti-windup & reset/5
  Gain/1 -> Discrete PI Controller with anti-windup & reset/1
  Gain1/1 -> V_ref/1
  Ki/1 -> Discrete PI Controller with anti-windup & reset/3
  Kp/1 -> Discrete PI Controller with anti-windup & reset/2

== system mcbdemo_28035_TARGET/Current_Controller/Control System/Close_Loop Control/Current_Controllers/PI_Controller_Iq ==
  I_ref : Inport
  I_fb : Inport  Port=2
  Data Store Read1 : DataStoreRead  DataStoreName=Enable  IndexOptions=Index vector (dialog)  Indices=1  OutputSizes=1
  Discrete PI Controller with anti-windup & reset : mcbcontrolslib/Discrete PI Controller  with anti-windup & reset  UpperSaturationLimit=0.9*Gain  LowerSaturationLimit=-0.9*Gain
      settings: SourceProductBaseCode=MT
  Gain : Gain  Gain=Gain  OutDataTypeStr=Inherit: Same as input
  Gain1 : Gain  Gain=1/Gain  OutDataTypeStr=Inherit: Same as input
  Ki : Constant  Value=0.0005  OutDataTypeStr=fixdt(1,32,24)  SampleTime=-1
  Kp : Constant  Value=0.25  OutDataTypeStr=fixdt(1,32,24)  SampleTime=-1
  Kp1 : Constant  Value=0  OutDataTypeStr=fixdt(1,32,24)  SampleTime=-1
  Logical Operator : Logic  Operator=NOT  IconShape=distinctive  AllPortsSameDT=off  OutDataTypeStr=boolean
  Sum : Sum  Inputs=|+-  OutDataTypeStr=Inherit: Same as first input
  V_ref : Outport  VectorParamsAs1DForOutWhenUnconnected=off
  wires:
  Discrete PI Controller with anti-windup & reset/1 -> Gain1/1
  Data Store Read1/1 -> Logical Operator/1
  I_fb/1 -> Sum/2
  I_ref/1 -> Sum/1
  Sum/1 -> Gain/1
  Logical Operator/1 -> Discrete PI Controller with anti-windup & reset/4
  Kp1/1 -> Discrete PI Controller with anti-windup & reset/5
  Gain1/1 -> V_ref/1
  Gain/1 -> Discrete PI Controller with anti-windup & reset/1
  Ki/1 -> Discrete PI Controller with anti-windup & reset/3
  Kp/1 -> Discrete PI Controller with anti-windup & reset/2

== system mcbdemo_28035_TARGET/Current_Controller/Input Scaling/Subsystem/Speed/speed cal ==
  Theta : Inport
  Add : Sum
  Gain : Gain  Gain=200  OutDataTypeStr=fixdt(1,32,15)
  Gain2 : Gain  Gain=0.9802  OutDataTypeStr=fixdt(1,32,15)
  Saturation : Saturate  UpperLimit=5  LowerLimit=-5
  Subtract : Sum  Inputs=+-
  Unit Delay : UnitDelay  SampleTime=-1  HasFrameUpgradeWarning=on
  Unit Delay1 : UnitDelay  SampleTime=-1  HasFrameUpgradeWarning=on
  Speed : Outport  VectorParamsAs1DForOutWhenUnconnected=off
  wires:
  Theta/1 -> Gain/1  "xk-1"
  Add/1 -> Speed/1, Unit Delay1/1  "yk"
  Unit Delay1/1 -> Gain2/1  "yk-1"
  Gain/1 -> Subtract/1, Unit Delay/1
  Unit Delay/1 -> Subtract/2
  Gain2/1 -> Add/2
  Subtract/1 -> Saturation/1
  Saturation/1 -> Add/1

== system mcbdemo_28035_TARGET/Current_Controller/Input Scaling/Subsystem/Speed/theta_unify ==
  raw_theta : Inport
  Add2 : Sum  Inputs=3  OutDataTypeStr=fixdt(1,32,15)
  Constant11 : Constant  Value=0  OutDataTypeStr=fixdt(1,32,15)
  Constant12 : Constant  Value=0  OutDataTypeStr=fixdt(1,32,15)
  Constant13 : Constant  Value=-1  OutDataTypeStr=fixdt(1,32,15)
  Constant9 : Constant  OutDataTypeStr=fixdt(1,32,15)
  Gain4 : Gain  Gain=-1  OutDataTypeStr=Inherit: Inherit via back propagation
  Switch1 : Switch
  Switch4 : Switch  Threshold=1
  unified_theta : Outport  VectorParamsAs1DForOutWhenUnconnected=off
  wires:
  Constant11/1 -> Switch4/3
  Switch1/1 -> Add2/1
  Gain4/1 -> Switch1/2
  raw_theta/1 -> Add2/2, Switch4/2, Gain4/1
  Constant12/1 -> Switch1/3
  Constant9/1 -> Switch1/1
  Switch4/1 -> Add2/3
  Constant13/1 -> Switch4/1
  Add2/1 -> unified_theta/1

== system mcbdemo_28035_TARGET/Current_Controller/SCI_TX(Code Generation)/SCI (Code Generation)/Data_Logging/Data ==
  Data : Inport
  Data_width : Inport  Port=2
  Action Port : ActionPort  ActionPortLabel=else
  Dummy : Constant  Value=hex2dec('0000')  OutDataTypeStr=uint32
  Mux : Mux  Inputs=2
  Data_out : Outport  VectorParamsAs1DForOutWhenUnconnected=off
  Iteration : Outport  Port=2  VectorParamsAs1DForOutWhenUnconnected=off
  wires:
  Data_width/1 -> Iteration/1
  Data/1 -> Mux/1
  Dummy/1 -> Mux/2
  Mux/1 -> Data_out/1

== system mcbdemo_28035_TARGET/Current_Controller/SCI_TX(Code Generation)/SCI (Code Generation)/Data_Logging/End ==
  Data : Inport
  Data_width : Inport  Port=2
  Action Port : ActionPort  ActionPortLabel=elseif(u1 == 99)
  Bias : Bias  Bias=1
  End : Constant  Value=hex2dec('45454545')  OutDataTypeStr=uint32
  Mux : Mux  Inputs=2
  Data_out : Outport  VectorParamsAs1DForOutWhenUnconnected=off
  Iteration : Outport  Port=2  VectorParamsAs1DForOutWhenUnconnected=off
  wires:
  Data/1 -> Mux/1
  Data_width/1 -> Bias/1
  Bias/1 -> Iteration/1
  End/1 -> Mux/2
  Mux/1 -> Data_out/1

== system mcbdemo_28035_TARGET/Current_Controller/SCI_TX(Code Generation)/SCI (Code Generation)/Data_Logging/Start ==
  Data : Inport
  Data_width : Inport  Port=2
  Action Port : ActionPort  ActionPortLabel=if(u1 == 0)
  Bias : Bias  Bias=1
  Mux : Mux  Inputs=2
  Start : Constant  Value=hex2dec('53535353')  OutDataTypeStr=uint32
  Data_out : Outport  VectorParamsAs1DForOutWhenUnconnected=off
  Iteration : Outport  Port=2  VectorParamsAs1DForOutWhenUnconnected=off
  wires:
  Data/1 -> Mux/2
  Data_width/1 -> Bias/1
  Bias/1 -> Iteration/1
  Start/1 -> Mux/1
  Mux/1 -> Data_out/1
